simulink model "cluster2"  (Simulink 7.1)
settings: Solver=FixedStepDiscrete  StartTime=0.0  StopTime=200  FixedStep=1  RelTol=1e-3
libraries: simulink x2
settings Model: Creator=vak  LastModifiedBy=vak
settings DebuggingCC: AlgebraicLoopMsg=none  ArtificialAlgebraicLoopMsg=none  SolverPrmCheckMsg=error  DiscreteInheritContinuousMsg=error

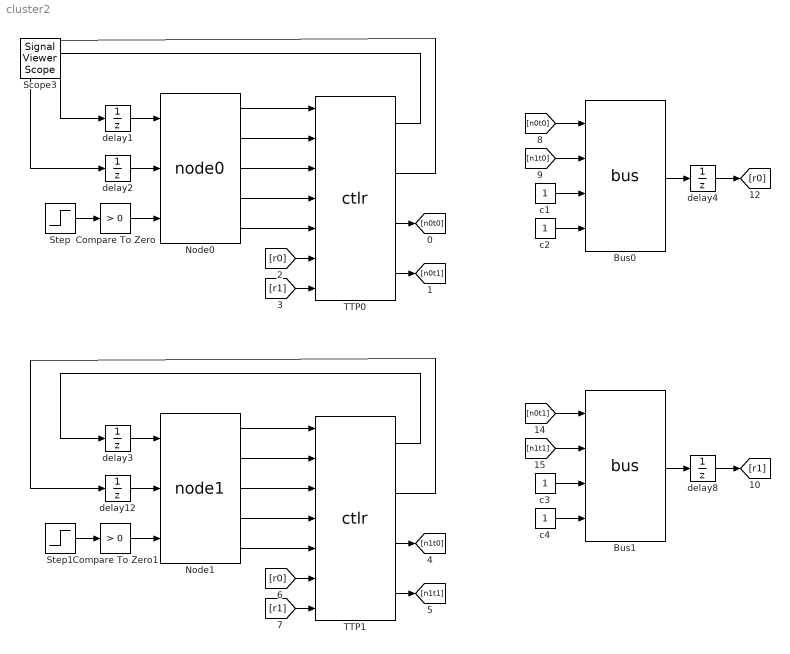
== system cluster2 ==
  Bus0 : S-Function  FunctionName=bus  SFunctionModules='bus-sfun bus'  EnableBusSupport=off
      mask Display:
      | port_label('input',1,'rn0')
      | port_label('input',2,'rn1')
      | port_label('input',3,'rn2')
      | port_label('input',4,'rn3')
      | port_label('output',1,'tx')
  Bus1 : S-Function  FunctionName=bus  SFunctionModules='bus-sfun bus'  EnableBusSupport=off
      mask Display:
      | port_label('input',1,'rn0')
      | port_label('input',2,'rn1')
      | port_label('input',3,'rn2')
      | port_label('input',4,'rn3')
      | port_label('output',1,'tx')
  Compare To Zero : simulink/Logic and Bit Operations/Compare To Zero  SystemSampleTime=-1  relop=>  LogicOutDataTypeMode=boolean  ZeroCross=off
  Compare To Zero1 : simulink/Logic and Bit Operations/Compare To Zero  SystemSampleTime=-1  relop=>  LogicOutDataTypeMode=boolean  ZeroCross=off
  Node0 : S-Function  FunctionName=node0  SFunctionModules='cpu-sfun node0'  EnableBusSupport=off
      mask Display: port_label('input',1,'datain')port_label('input',2,'ack')port_label('input',3,'rst')port_label('output',1,'dataout')port_label('output',2,'addr')port_label('output',3,'rd')port_label('output',4,'wrh')port_label('output',5,'wrl')
  Node1 : S-Function  FunctionName=node1  SFunctionModules='cpu-sfun node1'  EnableBusSupport=off
      mask Display: port_label('input',1,'datain')port_label('input',2,'ack')port_label('input',3,'rst')port_label('output',1,'dataout')port_label('output',2,'addr')port_label('output',3,'rd')port_label('output',4,'wrh')port_label('output',5,'wrl')
  Step : Step  Before=1  After=0  SampleTime=0  VectorParams1D=off
  Step1 : Step  Before=1  After=0  SampleTime=0  VectorParams1D=off
  TTP0 : S-Function  FunctionName=ctlr  SFunctionModules='ctlr-sfun ctlr'  EnableBusSupport=off
      mask Display:
      | port_label('input',1,'datain')
      | port_label('input',2,'addr')
      | port_label('input',3,'rd')
      | port_label('input',4,'wrh')
      | port_label('input',5,'wrl')
      | port_label('input',6,'rx0')
      | port_label('input',7,'rx1')
      | port_label('output',1,'dataout')
      | port_label('output',2,'ack')
      | port_label('output',3,'tx0')
      | port_label('output',4,'tx1')
  TTP1 : S-Function  FunctionName=ctlr  SFunctionModules='ctlr-sfun ctlr'  EnableBusSupport=off
      mask Display:
      | port_label('input',1,'datain')
      | port_label('input',2,'addr')
      | port_label('input',3,'rd')
      | port_label('input',4,'wrh')
      | port_label('input',5,'wrl')
      | port_label('input',6,'rx0')
      | port_label('input',7,'rx1')
      | port_label('output',1,'dataout')
      | port_label('output',2,'ack')
      | port_label('output',3,'tx0')
      | port_label('output',4,'tx1')
  c{1..4} (4 alike) : Constant  OutDataTypeMode=boolean  OutDataType=sfix(16)  OutScaling=2^0  OutDataTypeStr=boolean
  delay{1..4,8,12} (6 alike) : UnitDelay
  Scope3 : SignalViewerScope  IOType=viewer  RefreshTime=0.035000
  wires:
  Step/1 -> Compare To Zero/1
  TTP0/1 -> delay1/1
  TTP0/2 -> delay2/1
  delay1/1 -> Node0/1
  delay2/1 -> Node0/2
  TTP0/3 -> [n0t0]
  TTP0/4 -> [n0t1]
  [r0] -> TTP0/6
  [r1] -> TTP0/7
  Step1/1 -> Compare To Zero1/1
  TTP1/1 -> delay3/1
  TTP1/2 -> delay12/1
  delay3/1 -> Node1/1
  delay12/1 -> Node1/2
  TTP1/3 -> [n1t0]
  TTP1/4 -> [n1t1]
  [r0] -> TTP1/6
  [r1] -> TTP1/7
  [n0t0] -> Bus0/1
  [n1t0] -> Bus0/2
  c1/1 -> Bus0/3
  c2/1 -> Bus0/4
  [n0t1] -> Bus1/1
  [n1t1] -> Bus1/2
  c3/1 -> Bus1/3
  c4/1 -> Bus1/4
  Bus0/1 -> delay4/1
  delay4/1 -> [r0]
  Bus1/1 -> delay8/1
  delay8/1 -> [r1]
  Compare To Zero/1 -> Node0/3
  Node0/1 -> TTP0/1
  Node0/2 -> TTP0/2
  Node0/3 -> TTP0/3
  Node0/4 -> TTP0/4
  Node0/5 -> TTP0/5
  Compare To Zero1/1 -> Node1/3
  Node1/1 -> TTP1/1
  Node1/2 -> TTP1/2
  Node1/3 -> TTP1/3
  Node1/4 -> TTP1/4
  Node1/5 -> TTP1/5
